simulink model "task_1_scheme"  (R2024a)
settings: Solver=VariableStepAuto  StartTime=0.0  StopTime=10.0  RelTol=1e-3
settings Model: Creator=alexe  LastModifiedBy=alexe

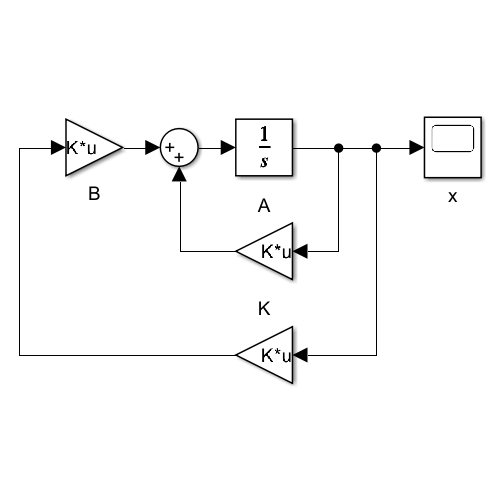
[thumbnail: Simulink's stored preview of the top-level diagram]
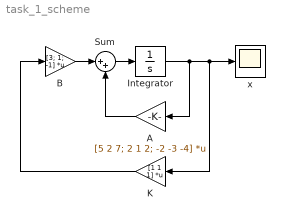
== system task_1_scheme ==
  A : Gain  Gain=[5 2 7; 2 1 2; -2 -3 -4]  Multiplication=Matrix(K*u)
  B : Gain  Gain=[3; 1; -1]  Multiplication=Matrix(K*u)
  Integrator : Integrator
  K : Gain  Gain=[1 1 1]  Multiplication=Matrix(K*u)
  Sum : Sum  Inputs=|++
  x : Scope
  wires:
  B/1 -> Sum/1
  Sum/1 -> Integrator/1
  A/1 -> Sum/2
  Integrator/1 -> A/1, K/1, x/1
  K/1 -> B/1
